simulink model "bary_source_seeking"  (Simulink 8.9)
settings: Solver=ode3  StartTime=0  StopTime=tf  FixedStep=1e-4  RelTol=1e-3
undefined symbols (not defined in the file): gaussianrnd, source_params, sys, x0, xhat0
settings Model: SuppressorTable=22 serialization::archive 11 0 6 0 0 0 11 0  Creator=brunolnetto  LastModifiedBy=brunolnetto
settings DataIOCC: LimitDataPoints=off  SaveFormat=Dataset  SignalLoggingSaveFormat=Dataset
settings DebuggingCC: UnderspecifiedInitializationDetection=Simplified  MergeDetectMultiDrivingBlocksExec=error  FcnCallInpInsideContextMsg=error  StateNameClashWarn=none  SFUnexpectedBacktrackingDiag=error  SFNoUnconditionalDefaultTransitionDiag=error
settings HardwareCC: ProdBitPerPointer=64  ProdLargestAtomicFloat=Float  ProdIntDivRoundTo=Zero  ProdEndianess=LittleEndian  ProdHWDeviceType=Specified
settings ModelReferenceCC: PropagateSignalLabelsOutOfModel=on
settings GRTTargetCC: TargetLangStandard=C99 (ISO)  GeneratePreprocessorConditionals=Use local settings  CombineOutputUpdateFcns=on  GRTInterface=off
settings ConfigComp: CovMetricSettings=dwe  CovHtmlReporting=off  CovSaveCumulativeToWorkspaceVar=off  CovSaveSingleToWorkspaceVar=off  CovExternalEMLEnable=on

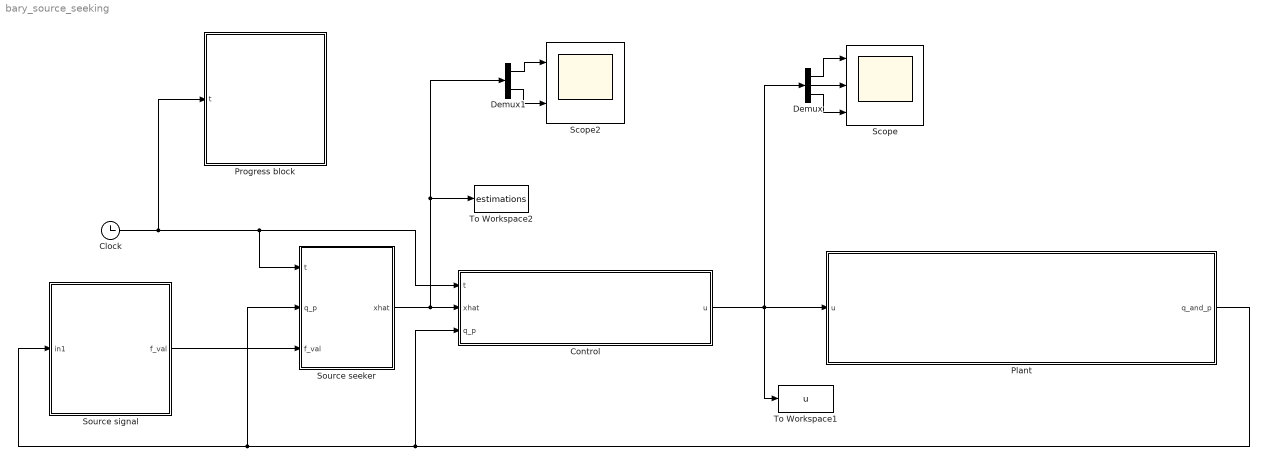
== system bary_source_seeking ==
  Clock : Clock
  Control : Subsystem
      mask Display: image('./controller.png');
  Demux : Demux  Outputs=3
  Demux1 : Demux  Outputs=2
  Plant : Subsystem
      mask Display: image('./plant.png');
  Progress block : MATLAB Function  TreatAsAtomicUnit=on
  Scope : Scope  NumInputPorts=3
  Scope2 : Scope  NumInputPorts=2
  Source seeker : Subsystem
  Source signal : MATLAB Function  TreatAsAtomicUnit=on
  To Workspace1 : ToWorkspace  VariableName=u  SaveFormat=Structure With Time  SampleTime=-1
  To Workspace2 : ToWorkspace  VariableName=estimations  SaveFormat=Structure With Time  SampleTime=-1
  wires:
  Clock/1 -> Progress block/1(t), Control/1(t), Source seeker/1(t)
  Source signal/1(f_val) -> Source seeker/3(f_val)
  Demux/2 -> Scope/2
  Demux/1 -> Scope/1
  Demux/3 -> Scope/3
  Source seeker/1(xhat) -> Control/2(xhat), Demux1/1, To Workspace2/1
  Demux1/2 -> Scope2/2
  Demux1/1 -> Scope2/1
  Plant/1(q_and_p) -> Control/3(q_p), Source seeker/2(q_p), Source signal/1(in1)
  Control/1(u) -> To Workspace1/1, Demux/1, Plant/1(u)

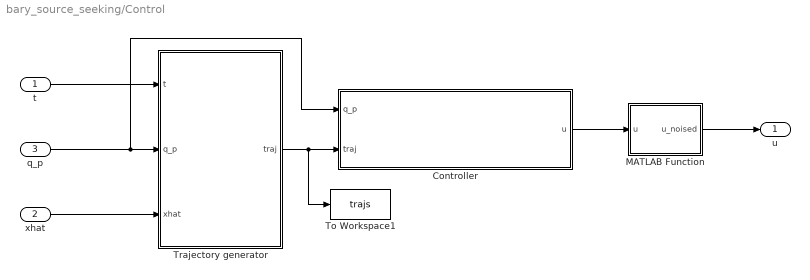
== system bary_source_seeking/Control ==
  t : Inport
  xhat : Inport  Port=2
  q_p : Inport  Port=3
  Controller : Subsystem
      mask Display: image('./controller.png');
  MATLAB Function : MATLAB Function  TreatAsAtomicUnit=on
  To Workspace1 : ToWorkspace  VariableName=trajs  SaveFormat=Structure With Time  SampleTime=-1
  Trajectory generator : Subsystem
  u : Outport
  wires:
  t/1 -> Trajectory generator/1(t)
  q_p/1 -> Controller/1(q_p), Trajectory generator/2(q_p)
  xhat/1 -> Trajectory generator/3(xhat)
  Trajectory generator/1(traj) -> To Workspace1/1, Controller/2(traj)
  Controller/1(u) -> MATLAB Function/1(u)
  MATLAB Function/1(u_noised) -> u/1

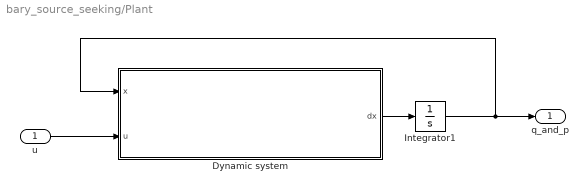
== system bary_source_seeking/Plant ==
  u : Inport
  Dynamic system : Subsystem
      mask Display: image('./plant.png')
  Integrator1 : Integrator  InitialCondition=x0
  q_and_p : Outport
  wires:
  Integrator1/1 -> q_and_p/1, Dynamic system/1(x)
  Dynamic system/1(dx) -> Integrator1/1
  u/1 -> Dynamic system/2(u)

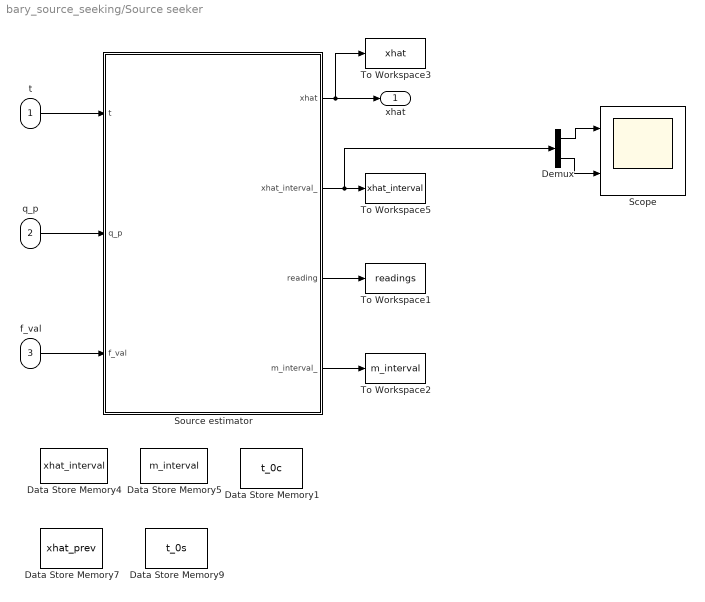
== system bary_source_seeking/Source seeker ==
  t : Inport
  q_p : Inport  Port=2
  f_val : Inport  Port=3
  Data Store Memory1 : DataStoreMemory  DataStoreName=t_0c  ShowAdditionalParam=off  OutDataTypeStr=double
  Data Store Memory4 : DataStoreMemory  DataStoreName=xhat_interval  InitialValue=xhat0  ShowAdditionalParam=off  OutDataTypeStr=double  Dimensions=[2, 1]
  Data Store Memory5 : DataStoreMemory  DataStoreName=m_interval  ShowAdditionalParam=off  OutDataTypeStr=double
  Data Store Memory7 : DataStoreMemory  DataStoreName=xhat_prev  InitialValue=xhat0 + gaussianrnd([0; 0], source_params.devval)  ShowAdditionalParam=off  OutDataTypeStr=double
  Data Store Memory9 : DataStoreMemory  DataStoreName=t_0s  ShowAdditionalParam=off  OutDataTypeStr=double
  Demux : Demux  Outputs=2
  Scope : Scope  NumInputPorts=2
  Source estimator : MATLAB Function  TreatAsAtomicUnit=on
  To Workspace1 : ToWorkspace  VariableName=readings  SaveFormat=Structure With Time  SampleTime=-1
  To Workspace2 : ToWorkspace  VariableName=m_interval  SaveFormat=Structure With Time  SampleTime=-1
  To Workspace3 : ToWorkspace  VariableName=xhat  SaveFormat=Structure With Time  SampleTime=-1
  To Workspace5 : ToWorkspace  VariableName=xhat_interval  SaveFormat=Structure With Time  SampleTime=-1
  xhat : Outport
  wires:
  Source estimator/1(xhat) -> xhat/1, To Workspace3/1
  t/1 -> Source estimator/1(t)
  q_p/1 -> Source estimator/2(q_p)
  f_val/1 -> Source estimator/3(f_val)
  Source estimator/2(xhat_interval_) -> Demux/1, To Workspace5/1
  Source estimator/3(reading) -> To Workspace1/1
  Source estimator/4(m_interval_) -> To Workspace2/1
  Demux/2 -> Scope/2
  Demux/1 -> Scope/1

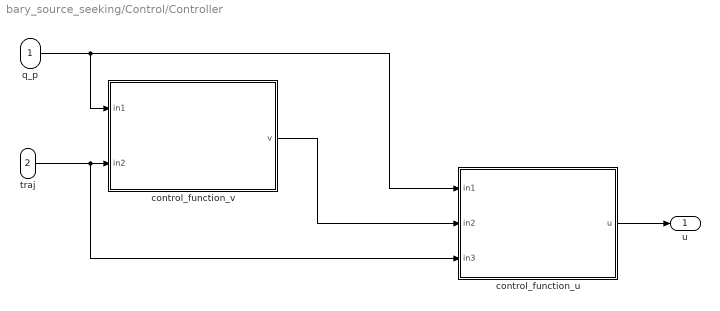
== system bary_source_seeking/Control/Controller ==
  q_p : Inport
  traj : Inport  Port=2
  control_function_u : MATLAB Function  TreatAsAtomicUnit=on
  control_function_v : MATLAB Function  TreatAsAtomicUnit=on
  u : Outport
  wires:
  control_function_v/1(v) -> control_function_u/2(in2)
  q_p/1 -> control_function_v/1(in1), control_function_u/1(in1)
  control_function_u/1(u) -> u/1
  traj/1 -> control_function_u/3(in3), control_function_v/2(in2)

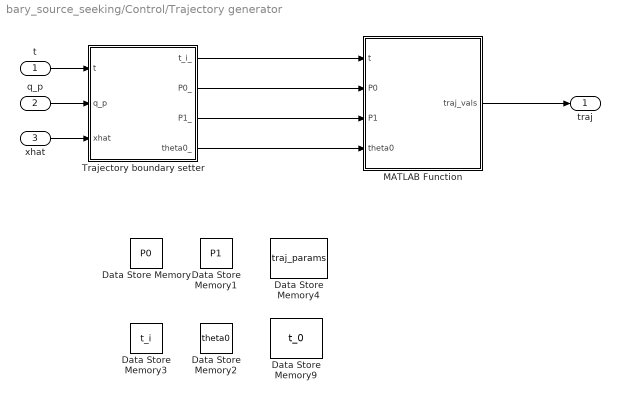
== system bary_source_seeking/Control/Trajectory generator ==
  t : Inport
  q_p : Inport  Port=2
  xhat : Inport  Port=3
  Data Store Memory : DataStoreMemory  DataStoreName=P0  WriteAfterWriteMsg=warning  WriteAfterReadMsg=warning  InitialValue=x0(1:2)  ShowAdditionalParam=off  OutDataTypeStr=double  Dimensions=[2, 1]
  Data Store Memory1 : DataStoreMemory  DataStoreName=P1  InitialValue=xhat0  ShowAdditionalParam=off  OutDataTypeStr=double
  Data Store Memory2 : DataStoreMemory  DataStoreName=theta0  InitialValue=x0(3)  ShowAdditionalParam=off  OutDataTypeStr=double
  Data Store Memory3 : DataStoreMemory  DataStoreName=t_i  ShowAdditionalParam=off  OutDataTypeStr=double
  Data Store Memory4 : DataStoreMemory  DataStoreName=traj_params  ShowAdditionalParam=off  OutDataTypeStr=double
  Data Store Memory9 : DataStoreMemory  DataStoreName=t_0  ShowAdditionalParam=off  OutDataTypeStr=double
  MATLAB Function : MATLAB Function  TreatAsAtomicUnit=on
  Trajectory boundary setter : MATLAB Function  TreatAsAtomicUnit=on
  traj : Outport
  wires:
  Trajectory boundary setter/4(theta0_) -> MATLAB Function/4(theta0)
  Trajectory boundary setter/2(P0_) -> MATLAB Function/2(P0)
  q_p/1 -> Trajectory boundary setter/2(q_p)
  MATLAB Function/1(traj_vals) -> traj/1
  t/1 -> Trajectory boundary setter/1(t)
  Trajectory boundary setter/1(t_i_) -> MATLAB Function/1(t)
  xhat/1 -> Trajectory boundary setter/3(xhat)
  Trajectory boundary setter/3(P1_) -> MATLAB Function/3(P1)

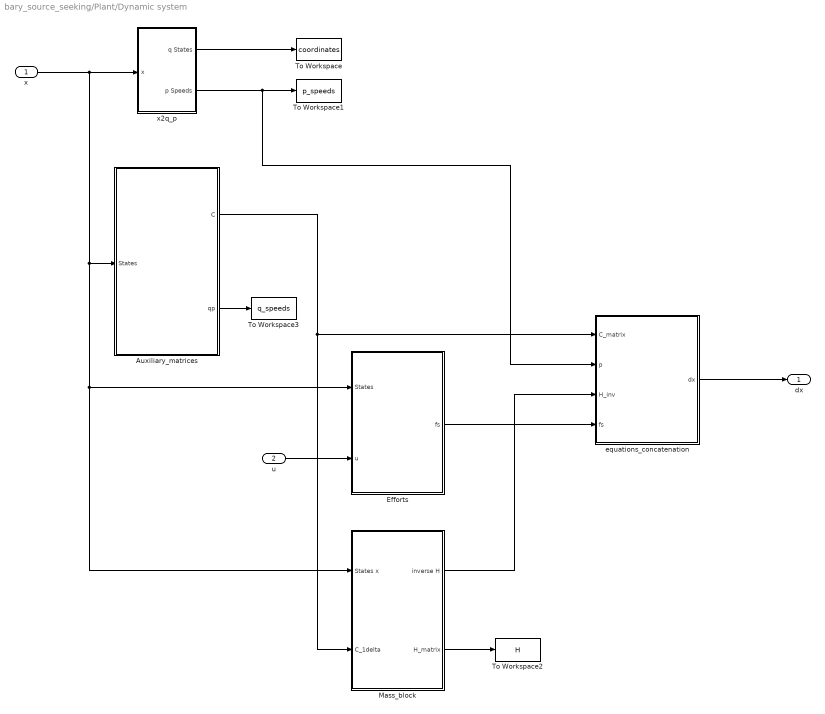
== system bary_source_seeking/Plant/Dynamic system ==
  x : Inport
  u : Inport  Port=2
  Auxiliary_matrices : Subsystem
  Efforts : Subsystem
  Mass_block : Subsystem
  To Workspace : ToWorkspace  VariableName=coordinates  SaveFormat=Structure With Time  SampleTime=-1
  To Workspace1 : ToWorkspace  VariableName=p_speeds  SaveFormat=Structure With Time  SampleTime=-1
  To Workspace2 : ToWorkspace  VariableName=H  SaveFormat=Structure With Time  SampleTime=-1
  To Workspace3 : ToWorkspace  VariableName=q_speeds  SaveFormat=Structure With Time  SampleTime=-1
  equations_concatenation : Subsystem
  x2q_p : Subsystem
  dx : Outport
  wires:
  Auxiliary_matrices/1(C) -> Mass_block/2("C_1delta  "), equations_concatenation/1(C_matrix)
  Auxiliary_matrices/2(qp) -> To Workspace3/1
  x2q_p/2(p Speeds) -> To Workspace1/1, equations_concatenation/2(p)
  x2q_p/1(q States) -> To Workspace/1
  Efforts/1(fs) -> equations_concatenation/4(fs)
  Mass_block/1(inverse H) -> equations_concatenation/3(H_inv)
  equations_concatenation/1(dx) -> dx/1
  u/1 -> Efforts/2(u)
  x/1 -> x2q_p/1(x), Efforts/1(States), Mass_block/1(States x), Auxiliary_matrices/1(States)
  Mass_block/2(H_matrix) -> To Workspace2/1

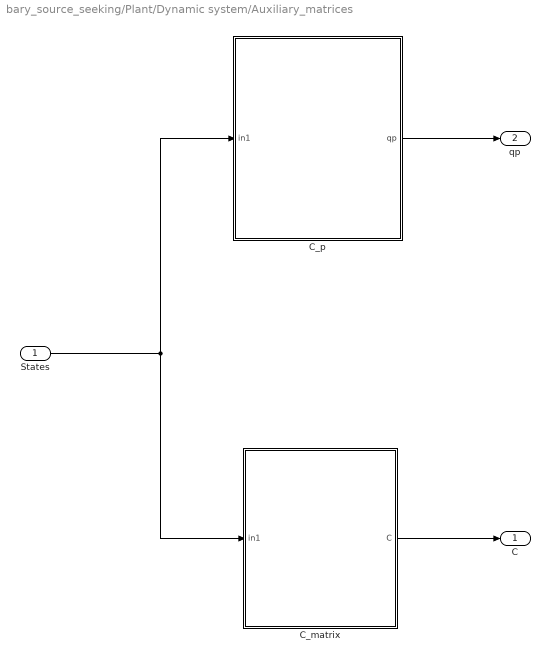
== system bary_source_seeking/Plant/Dynamic system/Auxiliary_matrices ==
  States : Inport
  C_matrix : MATLAB Function  TreatAsAtomicUnit=on
  C_p : MATLAB Function  TreatAsAtomicUnit=on
  C : Outport
  qp : Outport  Port=2
  wires:
  C_matrix/1(C) -> C/1
  States/1 -> C_p/1(in1), C_matrix/1(in1)
  C_p/1(qp) -> qp/1

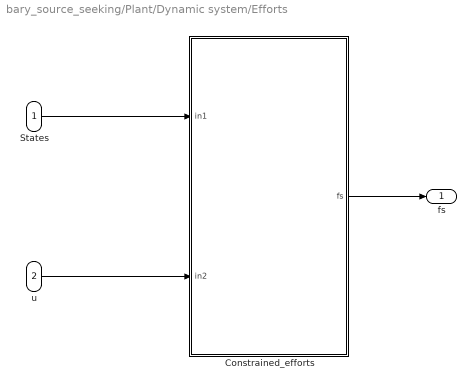
== system bary_source_seeking/Plant/Dynamic system/Efforts ==
  States : Inport
  u : Inport  Port=2
  Constrained_efforts : MATLAB Function  TreatAsAtomicUnit=on
  fs : Outport
  wires:
  States/1 -> Constrained_efforts/1(in1)
  u/1 -> Constrained_efforts/2(in2)
  Constrained_efforts/1(fs) -> fs/1

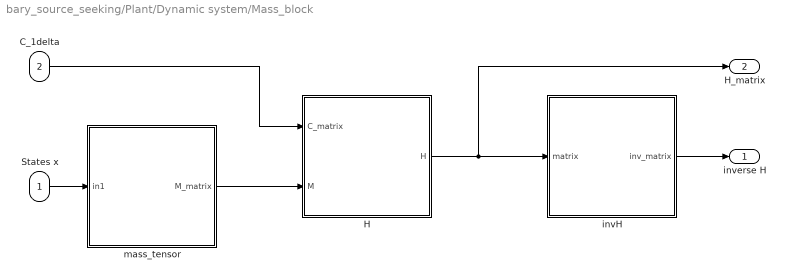
== system bary_source_seeking/Plant/Dynamic system/Mass_block ==
  States x : Inport
  "C_1delta  " : Inport  Port=2
  H : MATLAB Function  TreatAsAtomicUnit=on
  invH : MATLAB Function  TreatAsAtomicUnit=on
  mass_tensor : MATLAB Function  TreatAsAtomicUnit=on
  inverse H : Outport
  H_matrix : Outport  Port=2
  wires:
  States x/1 -> mass_tensor/1(in1)
  "C_1delta  "/1 -> H/1(C_matrix)
  invH/1(inv_matrix) -> inverse H/1
  H/1(H) -> invH/1(matrix), H_matrix/1
  mass_tensor/1(M_matrix) -> H/2(M)

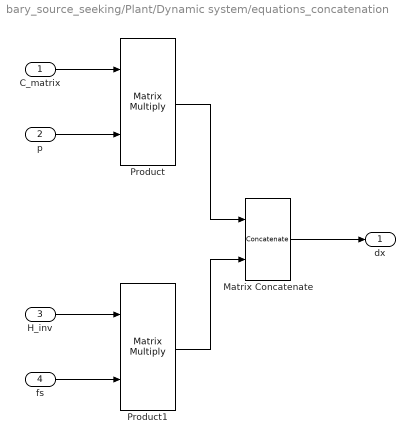
== system bary_source_seeking/Plant/Dynamic system/equations_concatenation ==
  C_matrix : Inport
  p : Inport  Port=2
  H_inv : Inport  Port=3
  fs : Inport  Port=4
  Matrix Concatenate : Concatenate  ConcatenateDimension=2
  Product : Product  Multiplication=Matrix(*)
  Product1 : Product  Multiplication=Matrix(*)
  dx : Outport
  wires:
  Product/1 -> Matrix Concatenate/1
  p/1 -> Product/2
  C_matrix/1 -> Product/1
  Product1/1 -> Matrix Concatenate/2
  H_inv/1 -> Product1/1
  fs/1 -> Product1/2
  Matrix Concatenate/1 -> dx/1

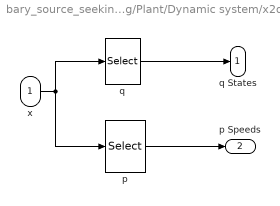
== system bary_source_seeking/Plant/Dynamic system/x2q_p ==
  x : Inport
  p : Selector  InputPortWidth=length(sys.kin.q) + length(sys.kin.p{end})  IndexOptions=Index vector (dialog)  Indices=(length(sys.kin.q))+1:(length(sys.kin.q) + length(sys.kin.p{end}))  OutputSizes=1
  q : Selector  InputPortWidth=length(sys.kin.q) + length(sys.kin.p{end})  IndexOptions=Index vector (dialog)  Indices=1:length(sys.kin.q)  OutputSizes=1
  q States : Outport
  p Speeds : Outport  Port=2
  wires:
  x/1 -> p/1, q/1
  q/1 -> q States/1
  p/1 -> p Speeds/1

== matlab function Control/Controller/control_function_u ==
  data: in1 input double; u output double; in2 input double; in3 input double
function u = ControlFunction_u(in1,in2,in3)

%    This function was generated by the Symbolic Math Toolbox version 7.2.

%    27-May-2022 11:27:43



p1 = in1(7,:);

p2 = in1(8,:);

p3 = in1(9,:);

phi1 = in1(4,:);

phi2 = in1(5,:);

phi3 = in1(6,:);

th = in1(3,:);

v1 = in2(1,:);

v2 = in2(2,:);

v3 = in2(3,:);

x = in1(1,:);

y = in1(2,:);

y1_ref = in3(1,:);

y2_ref = in3(4,:);

y3_ref = in3(7,:);

yp1_ref = in3(2,:);

yp2_ref = in3(5,:);

yp3_ref = in3(8,:);

ypp1_ref = in3(3,:);

ypp2_ref = in3(6,:);

ypp3_ref = in3(9,:);

t2 = th+5.235987755982989e-1;

t3 = th+1.047197551196598;

t4 = sin(t2);

t5 = sin(t3);

t6 = sin(phi1);

t7 = sin(phi2);

t8 = sin(phi3);

t9 = cos(t2);

t10 = t6.^2;

t11 = t10.*1.862411627770002e-9;

t12 = t7.^2;

t13 = t12.*1.862411627770002e-9;

t14 = t8.^2;

t15 = t14.*1.862411627770002e-9;

t16 = t11+t13+t15-1.044894955682166e-4;

t17 = 1.0./t16;

t18 = cos(t3);

t19 = cos(th);

t20 = sin(th);

t21 = cos(phi1);

t22 = cos(phi2);

t23 = cos(phi3);

t24 = p3.^2;

t25 = t4.*t5.*t17.*1.63236267389886e1;

t26 = t9.*t17.*t19.*1.63236267389886e1;

t27 = t17.*t18.*t20.*-1.63236267389886e1;

t28 = t5.*t17.*t19.*1.63236267389886e1;

t29 = t4.*t17.*t20.*1.63236267389886e1;

t30 = t9.*t17.*t18.*1.63236267389886e1;

t31 = t25+t26+t27+t28+t29+t30;

t32 = 1.0./t31;

t33 = p1.*-2.0e1;

t34 = x.*-1.0e2;

t35 = y1_ref.*1.0e2;

t36 = yp1_ref.*2.0e1;

t37 = t7.*t19.*t22.*t24.*6.008948770734595e-6;

t38 = t8.*t19.*t23.*t24.*-6.008948770734595e-6;

t39 = t6.*t20.*t21.*t24.*6.938536380660578e-6;

t40 = t7.*t20.*t22.*t24.*-3.469268190330289e-6;

t41 = t8.*t20.*t23.*t24.*-3.469268190330289e-6;

t42 = t33+t34+t35+t36+t37+t38+t39+t40+t41+v1+ypp1_ref;

t43 = t5.*t17.*5.924170616113744e-1;

t44 = p2.*-2.0e1;

t45 = y.*-1.0e2;

t46 = y2_ref.*1.0e2;

t47 = yp2_ref.*2.0e1;

t48 = t6.*t19.*t21.*t24.*-6.938536380660578e-6;

t49 = t7.*t19.*t22.*t24.*3.469268190330289e-6;

t50 = t8.*t19.*t23.*t24.*3.469268190330289e-6;

t51 = t7.*t20.*t22.*t24.*6.008948770734595e-6;

t52 = t8.*t20.*t23.*t24.*-6.008948770734595e-6;

t53 = t44+t45+t46+t47+t48+t49+t50+t51+t52+v2+ypp2_ref;

t54 = p3.*-2.0e1;

t55 = th.*-1.0e2;

t56 = y3_ref.*1.0e2;

t57 = yp3_ref.*2.0e1;

t58 = t21.^2;

t59 = t58.*1.164007267356251e62;

t60 = t22.^2;

t61 = t60.*1.164007267356251e62;

t62 = t23.^2;

t63 = t62.*1.164007267356251e62;

t64 = t59+t61+t63+6.530244270833333e66;

t65 = 1.0./t64;

t66 = phi1.*2.0;

t67 = sin(t66);

t68 = t24.*t67.*1.691871028134086e62;

t69 = phi2.*2.0;

t70 = sin(t69);

t71 = t24.*t70.*1.691871028134086e62;

t72 = phi3.*2.0;

t73 = sin(t72);

t74 = t24.*t73.*1.691871028134086e62;

t75 = t24.*3.926713624160408e26;

t76 = p2.*p3.*t6.*t19.*t21.*2.706993645014537e63;

t77 = p1.*p3.*t7.*t19.*t22.*-2.344325264465624e63;

t78 = p2.*p3.*t7.*t19.*t22.*-1.353496822507269e63;

t79 = p1.*p3.*t8.*t19.*t23.*2.344325264465624e63;

t80 = p2.*p3.*t8.*t19.*t23.*-1.353496822507269e63;

t81 = p1.*p3.*t6.*t20.*t21.*-2.706993645014537e63;

t82 = p1.*p3.*t7.*t20.*t22.*1.353496822507269e63;

t83 = p2.*p3.*t7.*t20.*t22.*-2.344325264465624e63;

t84 = p1.*p3.*t8.*t20.*t23.*1.353496822507269e63;

t85 = p2.*p3.*t8.*t20.*t23.*2.344325264465624e63;

t86 = t68+t71+t74+t75+t76+t77+t78+t79+t80+t81+t82+t83+t84+t85;

t87 = t65.*t86.*1.0;

t88 = t54+t55+t56+t57+t87+v3+ypp3_ref;

t89 = t9.*t17.*5.924170616113744e-1;

t90 = t4.*t17.*5.924170616113744e-1;

t91 = t17.*t19.*5.924170616113744e-1;

u = [t32.*t53.*(t43+t89).*-1.0+t32.*t42.*(t90-t17.*t18.*5.924170616113744e-1).*1.0+t32.*t88.*(t4.*t5.*7.592384529762141e2+t9.*t18.*7.592384529762141e2);t32.*t53.*(t43+t17.*t20.*5.924170616113744e-1)+t32.*t42.*(t91+t17.*t18.*5.924170616113744e-1)+t32.*t88.*(t5.*t19.*7.592384529762141e2-t18.*t20.*7.592384529762141e2);t32.*t42.*(t90+t91).*-1.0+t32.*t53.*(t89-t17.*t20.*5.924170616113744e-1)+t32.*t88.*(t4.*t20.*7.592384529762141e2+t9.*t19.*7.592384529762141e2)];

end

== matlab function Control/Trajectory generator/MATLAB Function ==
  data: t input double; traj_vals output double; P0 input double; P1 input double; theta0 input double; trajectory_info parameter double; t_0 data_store_memory double
function traj_vals = traj_gen(t, P0, P1, theta0, trajectory_info)
    % Origin and destiny
    P0 = double(P0);
    P1 = double(P1);    
    
    if(trajectory_info.is_dest_noised)
        sP = trajectory_info.devval_P0;
        zP = gaussianrnd([0; 0], sP);
        P1 = P1 + zP;
    end
    
    % Trajectory options
    T = trajectory_info.T_traj;
    deltas = trajectory_info.deltas;
    
    delta_x = deltas(1);
    delta_y = deltas(2);
    delta_th = deltas(3);
    
    x_y = P0 + t*(P1 - P0)/T;
    
    if(trajectory_info.is_traj_noised)
        s0 = trajectory_info.devval_traj;
        z0 = gaussianrnd([0; 0], s0);
        x_y = x_y + z0;
    end
    
    dx_y = (P1 - P0)/T;
    th = atan2(dx_y(2), dx_y(1));
    
    traj_vals = [x_y(1); dx_y(1); 0; ...
                 x_y(2); dx_y(2); 0; ...
                 th; 0; 0];
end

== matlab function Source seeker/Source estimator ==
  settings: updateMethod=DISCRETE  sampleTime=1e-4
  data: t input double; q_p input double; xhat_interval data_store_memory double; m_interval data_store_memory double; xhat_prev data_store_memory double; t_0c data_store_memory double; f_val input double; xhat output double; xhat_interval_ output double; reading output double; source_params parameter double; m_interval_ output double; t_0s data_store_memory double

function [xhat, xhat_interval_, reading, m_interval_] = ...
            source_estimation(t, q_p, f_val, ...
                              source_params)
    global t_0c t_0s xhat_prev m_interval xhat_interval;
    
    % Source seeking parameters
    nu = source_params.nu;
    lambda = source_params.lambda;
    T_cur = source_params.T_cur;
    T_sample = source_params.T_sample;
    devval = source_params.devval;
    
    % Current position
    x_curr = q_p(1:2, 1);
    
    n = length(x_curr);
    
    % Update source estimation window
    if(t - t_0c > T_cur)
        t_0c = t;
        
        z = gaussianrnd([0; 0], devval);
        xhat_prev = xhat_interval + z;
    
    elseif(t - t_0s > T_sample)
        t_0s = t;
        
        % Barycenter along the trajectory
        e_i = exp(-nu*f_val);
        
        bary_num = lambda*m_interval*xhat_interval + e_i*x_curr;
        bary_den = lambda*m_interval + e_i;
        
        xhat_interval = bary_num/bary_den;
        m_interval = bary_den;
    
    end
    
    xhat = xhat_prev;
    xhat_interval_ = xhat_interval;
    m_interval_ = m_interval;
    reading = f_val;
end

== matlab function Control/Trajectory generator/Trajectory boundary setter ==
  settings: updateMethod=DISCRETE  sampleTime=1e-4
  data: t_i_ output double; P0_ output double; P1_ output double; theta0_ output double; t input double; q_p input double; xhat input double; t_0 data_store_memory double; P0 data_store_memory double; P1 data_store_memory double; theta0 data_store_memory double; source_params parameter double
function [t_i_, P0_, P1_, theta0_] = trajectory(t, q_p, xhat, source_params)
    global P0 P1 t_0 theta0;
    
    T_cur = source_params.T_cur;
    
    % Initial and end trajectory points
    if(t - t_0 > T_cur)
        t_0 = t;
        
%         P0 = q_p(1:2);
%         P1 = xhat;

        P0 = P1;
        P1 = xhat;

        theta0 = q_p(3);
        
        t_i = t - t_0;
    end
    
    % Save state points
    P0_ = P0;
    P1_ = P1;
    theta0_ = theta0;
    t_i_ = t - t_0;
end

== matlab function Control/Controller/control_function_v ==
  data: in1 input double; v output double; in2 input double
function v = ControlFunction_v(in1,in2)

%    This function was generated by the Symbolic Math Toolbox version 7.2.

%    27-May-2022 11:27:43



p1 = in1(7,:);

p2 = in1(8,:);

p3 = in1(9,:);

th = in1(3,:);

x = in1(1,:);

y = in1(2,:);

y1_ref = in2(1,:);

y2_ref = in2(4,:);

y3_ref = in2(7,:);

yp1_ref = in2(2,:);

yp2_ref = in2(5,:);

yp3_ref = in2(8,:);

v = [p1.*-1.972066529187303e1+p2.*2.479096856783359e-14-p3.*4.22968703690907e-13-th.*8.523067115214349e-12-x.*2.943354051375265e2+y.*4.933795829235421e-13+y1_ref.*2.943354051375265e2-y2_ref.*4.933795829235421e-13+y3_ref.*8.523067115214349e-12+yp1_ref.*1.972066529187303e1-yp2_ref.*2.479096856783359e-14+yp3_ref.*4.22968703690907e-13;p1.*1.074138943653674e-14-p2.*1.980221538871086e1+p3.*4.166737848583495e-25+th.*8.387311679532198e-24+x.*2.137773955712297e-13-y.*2.9602763395128e2-y1_ref.*2.137773955712297e-13+y2_ref.*2.9602763395128e2-y3_ref.*8.387311679532198e-24-yp1_ref.*1.074138943653674e-14+yp2_ref.*1.980221538871086e1-yp3_ref.*4.166737848583495e-25;p1.*-4.94891936152957e-13+p2.*1.136209469416926e-24-p3.*2.047431043082865e1-th.*3.095256494049752e2-x.*9.380271259297049e-12+y.*2.265754980731487e-23+y1_ref.*9.380271259297049e-12-y2_ref.*2.265754980731487e-23+y3_ref.*3.095256494049752e2+yp1_ref.*4.94891936152957e-13-yp2_ref.*1.136209469416926e-24+yp3_ref.*2.047431043082865e1];

end

== matlab function Control/MATLAB Function ==
  settings: updateMethod=DISCRETE  sampleTime=1e-4
  data: u input double; u_noised output double; control_info parameter double
function u_noised = fcn(u, control_info)
    if(control_info.is_control_noised)
        su = control_info.devval;
        
        nu = length(u);
        zero_u = zeros(nu, 1);
        zu = gaussianrnd(zero_u, su);
        
        u_noised = u + zu;
    else
        u_noised = u;
    end
end

== matlab function Source signal ==
  data: in1 input double; f_val output double
function f_val = source_signal(in1)

%    This function was generated by the Symbolic Math Toolbox version 8.1.

%    14-Sep-2021 13:02:23



x = in1(1,:);

y = in1(2,:);

f_val = x.^2+y.^2;

end

== matlab function Plant/Dynamic system/Auxiliary_matrices/C_matrix ==
  data: in1 input double; C output double
function C = ConstraintMatrix(in1)

%    This function was generated by the Symbolic Math Toolbox version 7.2.

%    27-May-2022 11:27:32



th = in1(3,:);

t2 = cos(th);

t3 = sin(th);

t4 = t3.*-5.813953488372093;

t5 = t2.*5.813953488372093;

C = reshape([1.0,0.0,0.0,t3.*1.162790697674419e1,t2.*1.007006283470277e1+t4,t2.*-1.007006283470277e1+t4,0.0,1.0,0.0,t2.*-1.162790697674419e1,t3.*1.007006283470277e1+t5,t3.*-1.007006283470277e1+t5,0.0,0.0,1.0,-2.906976744186047,-2.906976744186047,-2.906976744186047],[6,3]);

end

== matlab function Plant/Dynamic system/Efforts/Constrained_efforts ==
  data: in1 input double; fs output double; in2 input double
function fs = ConstrainedEffort(in1,in2)

%    This function was generated by the Symbolic Math Toolbox version 7.2.

%    27-May-2022 11:27:32



p1 = in1(7,:);

p2 = in1(8,:);

p3 = in1(9,:);

phi1 = in1(4,:);

phi2 = in1(5,:);

phi3 = in1(6,:);

tau1 = in2(1,:);

tau2 = in2(2,:);

tau3 = in2(3,:);

th = in1(3,:);

t2 = cos(th);

t3 = sin(th);

t4 = p3.^2;

t5 = cos(phi2);

t6 = sin(phi2);

t7 = cos(phi3);

t8 = sin(phi3);

t9 = cos(phi1);

t10 = sin(phi1);

fs = [t2.*tau2.*1.007006283470277e1+t3.*tau1.*1.162790697674419e1-t2.*tau3.*1.007006283470277e1-t3.*tau2.*5.813953488372093-t3.*tau3.*5.813953488372093-t2.*t4.*t5.*t6.*2.535776381249999e-6+t3.*t4.*t5.*t6.*1.464031176319382e-6+t2.*t4.*t7.*t8.*2.535776381249999e-6+t3.*t4.*t7.*t8.*1.464031176319382e-6-t3.*t4.*t9.*t10.*2.928062352638764e-6;t2.*tau1.*-1.162790697674419e1+t2.*tau2.*5.813953488372093+t2.*tau3.*5.813953488372093+t3.*tau2.*1.007006283470277e1-t3.*tau3.*1.007006283470277e1-t2.*t4.*t5.*t6.*1.464031176319382e-6-t3.*t4.*t5.*t6.*2.535776381249999e-6-t2.*t4.*t7.*t8.*1.464031176319382e-6+t3.*t4.*t7.*t8.*2.535776381249999e-6+t2.*t4.*t9.*t10.*2.928062352638764e-6;tau1.*-2.906976744186047-tau2.*2.906976744186047-tau3.*2.906976744186047-t2.*t3.*t4.*1.434929627468613e-42-t4.*t5.*t6.*7.32015588159691e-7-t4.*t7.*t8.*7.32015588159691e-7-t4.*t9.*t10.*7.32015588159691e-7+p1.*p3.*t2.*t5.*t6.*5.071552762499998e-6-p1.*p3.*t3.*t5.*t6.*2.928062352638764e-6+p2.*p3.*t2.*t5.*t6.*2.928062352638764e-6+p2.*p3.*t3.*t5.*t6.*5.071552762499998e-6-p1.*p3.*t2.*t7.*t8.*5.071552762499998e-6-p1.*p3.*t3.*t7.*t8.*2.928062352638764e-6+p2.*p3.*t2.*t7.*t8.*2.928062352638764e-6-p2.*p3.*t3.*t7.*t8.*5.071552762499998e-6+p1.*p3.*t3.*t9.*t10.*5.856124705277528e-6-p2.*p3.*t2.*t9.*t10.*5.856124705277528e-6];

end

== matlab function Plant/Dynamic system/Mass_block/H ==
  data: C_matrix input double; H output double; M input double
function H = ConstrinedMassMatrix(C_matrix, M)
% MASSMATRIX
%    This function was generated by the Symbolic Math Toolbox version 7.2.
%    16-Oct-2020 11:55:07

    H = C_matrix'*M*C_matrix;
end

== matlab function Plant/Dynamic system/Mass_block/mass_tensor ==
  data: in1 input double; M_matrix output double
function M_matrix = Mass_matrix(in1)

%    This function was generated by the Symbolic Math Toolbox version 7.2.

%    27-May-2022 11:27:32



phi1 = in1(4,:);

phi2 = in1(5,:);

phi3 = in1(6,:);

th = in1(3,:);

t2 = cos(phi1);

t3 = cos(phi2);

t4 = cos(phi3);

t5 = cos(th);

t6 = sin(th);

M_matrix = reshape([4.22e-1,0.0,0.0,0.0,0.0,0.0,0.0,4.22e-1,0.0,0.0,0.0,0.0,0.0,0.0,t2.^2.*2.518133623269337e-7+t3.^2.*2.518133623269337e-7+t4.^2.*2.518133623269337e-7+t5.^2.*1.3875e-2+t6.^2.*1.3875e-2+2.520833333333333e-4,0.0,0.0,0.0,0.0,0.0,0.0,0.0,0.0,0.0,0.0,0.0,0.0,0.0,0.0,0.0,0.0,0.0,0.0,0.0,0.0,0.0],[6,6]);

end

== matlab function Plant/Dynamic system/Mass_block/invH ==
  data: matrix input double; inv_matrix output double
function inv_matrix = matrix_inverse(matrix)
% MASSMATRIX
%    This function was generated by the Symbolic Math Toolbox version 7.2.
%    16-Oct-2020 11:55:07

    inv_matrix = inv(matrix);
end

== matlab function Progress block ==
  data: t input double; tf parameter double
function progress_block(t, tf)
    coder.extrinsic('num2str');
    disp(['(', num2str(tf), ',', num2str(t), ',', num2str(100*t/tf), ')']);
end

== matlab function Plant/Dynamic system/Auxiliary_matrices/C_p ==
  data: in1 input double; qp output double
function qp = KinematicVector(in1)

%    This function was generated by the Symbolic Math Toolbox version 7.2.

%    27-May-2022 11:27:31



p1 = in1(7,:);

p2 = in1(8,:);

p3 = in1(9,:);

th = in1(3,:);

t2 = p3.*-2.906976744186047;

t3 = cos(th);

t4 = sin(th);

t5 = p2.*t3.*5.813953488372093;

t6 = p1.*t4.*-5.813953488372093;

qp = [p1;p2;p3;t2+p1.*t4.*1.162790697674419e1-p2.*t3.*1.162790697674419e1;t2+t5+t6+p1.*t3.*1.007006283470277e1+p2.*t4.*1.007006283470277e1;t2+t5+t6-p1.*t3.*1.007006283470277e1-p2.*t4.*1.007006283470277e1];

end
